simulink model "eco"  (Simulink 7.2)
settings: Solver=ode45  StartTime=0.0  StopTime=10.0  RelTol=1e-3
libraries: dspsigops x1, dspsrcs4 x1, dspsnks4 x1
settings Model: Creator=Gus  LastModifiedBy=Gus

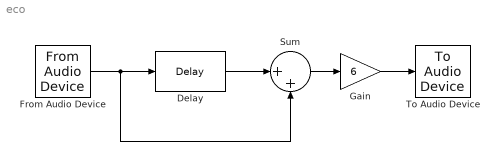
== system eco ==
  Delay : dspsigops/Delay  dly_unit=Samples  delay=44100*5  ic_detail=off  dif_ic_for_ch=off  dif_ic_for_dly=off  ic=0  reset_popup=None
  From Audio Device : dspsrcs4/From Audio Device  DialogController=dspDDGCreate  DialogControllerArgs=DataTag0  deviceName=Default  numChannels=2  sampleRate=44100  deviceDatatype=Determine from output data type  autoBufferSize=on  bufferSize=4096  queueDuration=1.0  frameSize=1024  outputDatatype=single
  Gain : Gain  Gain=6  ParameterDataType=sfix(16)  ParameterScaling=2^0  OutDataType=sfix(16)  OutScaling=2^0
  Sum : Sum  Inputs=|++  OutDataType=sfix(16)  OutScaling=2^0
  To Audio Device : dspsnks4/To Audio Device  DialogController=dspDDGCreate  DialogControllerArgs=DataTag1  deviceName=Default  inheritSampleRate=on  sampleRate=44100  deviceDatatype=Determine from input data type  autoBufferSize=on  bufferSize=4096  queueDuration=1.0
  wires:
  From Audio Device/1 -> Delay/1, Sum/2
  Sum/1 -> Gain/1
  Delay/1 -> Sum/1
  Gain/1 -> To Audio Device/1
